simulink model "gm_hybrid_lht_vnl"  (R2019b)
settings: Solver=FixedStepDiscrete  StartTime=0.0  StopTime=inf  FixedStep=1/120e6  RelTol=1e-3
undefined symbols (not defined in the file or in its folder): bt, height, nTheta, width
libraries: hdlsllib x632, simulink x518, hdlmdlgenlib x7, dspsrcs4 x1
(part 7 of 18)

== system gm_hybrid_lht_vnl/Hybrid LHT/Hybrid LHT Accumulator/Accumulator with Switches/Accumulator_instance7 ==
  shift : Inport  OutDataTypeStr=fixdt(0, 6, 0)  PortDimensions=1  SampleTime=8.33333333333333e-09
  mode : Inport  Port=2  OutDataTypeStr=boolean  PortDimensions=1  SampleTime=8.33333333333333e-09
  address : Inport  Port=3  OutDataTypeStr=fixdt(0, 11, 0)  PortDimensions=1  SampleTime=8.33333333333333e-09
  edge : Inport  Port=4  OutDataTypeStr=boolean  PortDimensions=1  SampleTime=8.33333333333333e-09
  AND : Logic  IconShape=distinctive  AllPortsSameDT=off  OutDataTypeStr=boolean
  Add : Sum  OutDataTypeStr=fixdt(0, ceil(log2(maxRho*2)), 0)
  Bit Concat : hdlsllib/Logic and Bit Operations/Bit Concat  numInputs=2
      settings: SourceProductName=Simulink
  Bit Slice : hdlsllib/Logic and Bit Operations/Bit Slice  lidx=voteWL-1  ridx=0
  Bitwise AND : simulink/Logic and Bit Operations/Bitwise Operator  logicop=AND  UseBitMask=off  NumInputPorts=2  BitMask=bin2dec('11011001')  BitMaskRealWorld=Stored Integer
  Bitwise NOT : simulink/Logic and Bit Operations/Bitwise Operator  logicop=NOT  UseBitMask=off  BitMask=bin2dec('11011001')  BitMaskRealWorld=Stored Integer
  Bitwise OR : simulink/Logic and Bit Operations/Bitwise Operator  logicop=OR  UseBitMask=off  NumInputPorts=2  BitMask=bin2dec('11011001')  BitMaskRealWorld=Stored Integer
  Block RAM : Subsystem
  Constant : Constant  Value=0  OutDataTypeStr=fixdt(0, 36-voteWL, 0)  SampleTime=-1
  Constant1 : Constant  Value=2^(voteWL)-1  OutDataTypeStr=fixdt(0, 36, 0)  SampleTime=-1
  Delay{,1..2,4..5} (5 alike) : Delay  DelayLength=1
  Multiport Switch : MultiPortSwitch  DataPortOrder=Zero-based contiguous  Inputs=2  zeroidx=on
  Multiport Switch1 : MultiPortSwitch  DataPortOrder=Zero-based contiguous  Inputs=2  zeroidx=on
  Relational Operator : RelationalOperator  Operator===  OutDataTypeStr=boolean  RndMeth=Simplest
  Shift Arithmetic : ArithShift  BitShiftNumberSource=Input port  BitShiftNumber=8  BitShiftDirection=Left  DiagnosticForOORShift=Error
      settings: InputPortMap=u0,p1
  Shift Arithmetic1 : ArithShift  BitShiftNumberSource=Input port  BitShiftNumber=8  BitShiftDirection=Left  DiagnosticForOORShift=Error
      settings: InputPortMap=u0,p1
  Shift Arithmetic2 : ArithShift  BitShiftNumberSource=Input port  BitShiftNumber=8  BitShiftDirection=Right  DiagnosticForOORShift=Error
      settings: InputPortMap=u0,p1
  Signal Specification : SignalSpecification  OutDataTypeStr=fixdt(0, 36, 0)
  Vote : Constant  OutDataTypeStr=fixdt(0,1,0)  SampleTime=-1
  Zero : Constant  Value=0  OutDataTypeStr=fixdt(0,1,0)  SampleTime=-1
  hps : Outport
  wires:
  Zero/1 -> Multiport Switch/2
  Vote/1 -> Add/1
  Shift Arithmetic1/1 -> Bitwise NOT/1
  Relational Operator/1 -> AND/2
  Delay4/1 -> Shift Arithmetic1/2, Shift Arithmetic/2, Shift Arithmetic2/2
  Delay2/1 -> Multiport Switch1/1
  Delay1/1 -> AND/1, Block RAM/3(wr_en)
  Delay/1 -> Relational Operator/1, Block RAM/2(wr_addr)
  Constant1/1 -> Shift Arithmetic1/1
  Constant/1 -> Bit Concat/1
  Bitwise NOT/1 -> Bitwise AND/1
  Bit Slice/1 -> hps/1, Add/2
  AND/1 -> Delay2/1
  shift/1 -> Delay4/1
  mode/1 -> Multiport Switch/1
  address/1 -> Relational Operator/2, Delay/1, Block RAM/4(rd_addr)
  edge/1 -> Delay1/1
  Delay5/1 -> Multiport Switch1/3
  Shift Arithmetic/1 -> Bitwise OR/2
  Bit Concat/1 -> Shift Arithmetic/1
  Multiport Switch/1 -> Bit Concat/2
  Add/1 -> Multiport Switch/3
  Shift Arithmetic2/1 -> Bit Slice/1
  Bitwise AND/1 -> Bitwise OR/1
  Bitwise OR/1 -> Delay5/1, Block RAM/1(wr_data)
  Signal Specification/1 -> Multiport Switch1/2
  Multiport Switch1/1 -> Bitwise AND/2, Shift Arithmetic2/1
  Block RAM/1(rd_data) -> Signal Specification/1

== system gm_hybrid_lht_vnl/Hybrid LHT/Hybrid LHT Accumulator/Accumulator with Switches/Accumulator_instance8 ==
  shift : Inport  OutDataTypeStr=fixdt(0, 6, 0)  PortDimensions=1  SampleTime=8.33333333333333e-09
  mode : Inport  Port=2  OutDataTypeStr=boolean  PortDimensions=1  SampleTime=8.33333333333333e-09
  address : Inport  Port=3  OutDataTypeStr=fixdt(0, 11, 0)  PortDimensions=1  SampleTime=8.33333333333333e-09
  edge : Inport  Port=4  OutDataTypeStr=boolean  PortDimensions=1  SampleTime=8.33333333333333e-09
  AND : Logic  IconShape=distinctive  AllPortsSameDT=off  OutDataTypeStr=boolean
  Add : Sum  OutDataTypeStr=fixdt(0, ceil(log2(maxRho*2)), 0)
  Bit Concat : hdlsllib/Logic and Bit Operations/Bit Concat  numInputs=2
      settings: SourceProductName=Simulink
  Bit Slice : hdlsllib/Logic and Bit Operations/Bit Slice  lidx=voteWL-1  ridx=0
  Bitwise AND : simulink/Logic and Bit Operations/Bitwise Operator  logicop=AND  UseBitMask=off  NumInputPorts=2  BitMask=bin2dec('11011001')  BitMaskRealWorld=Stored Integer
  Bitwise NOT : simulink/Logic and Bit Operations/Bitwise Operator  logicop=NOT  UseBitMask=off  BitMask=bin2dec('11011001')  BitMaskRealWorld=Stored Integer
  Bitwise OR : simulink/Logic and Bit Operations/Bitwise Operator  logicop=OR  UseBitMask=off  NumInputPorts=2  BitMask=bin2dec('11011001')  BitMaskRealWorld=Stored Integer
  Block RAM : Subsystem
  Constant : Constant  Value=0  OutDataTypeStr=fixdt(0, 36-voteWL, 0)  SampleTime=-1
  Constant1 : Constant  Value=2^(voteWL)-1  OutDataTypeStr=fixdt(0, 36, 0)  SampleTime=-1
  Delay{,1..2,4..5} (5 alike) : Delay  DelayLength=1
  Multiport Switch : MultiPortSwitch  DataPortOrder=Zero-based contiguous  Inputs=2  zeroidx=on
  Multiport Switch1 : MultiPortSwitch  DataPortOrder=Zero-based contiguous  Inputs=2  zeroidx=on
  Relational Operator : RelationalOperator  Operator===  OutDataTypeStr=boolean  RndMeth=Simplest
  Shift Arithmetic : ArithShift  BitShiftNumberSource=Input port  BitShiftNumber=8  BitShiftDirection=Left  DiagnosticForOORShift=Error
      settings: InputPortMap=u0,p1
  Shift Arithmetic1 : ArithShift  BitShiftNumberSource=Input port  BitShiftNumber=8  BitShiftDirection=Left  DiagnosticForOORShift=Error
      settings: InputPortMap=u0,p1
  Shift Arithmetic2 : ArithShift  BitShiftNumberSource=Input port  BitShiftNumber=8  BitShiftDirection=Right  DiagnosticForOORShift=Error
      settings: InputPortMap=u0,p1
  Signal Specification : SignalSpecification  OutDataTypeStr=fixdt(0, 36, 0)
  Vote : Constant  OutDataTypeStr=fixdt(0,1,0)  SampleTime=-1
  Zero : Constant  Value=0  OutDataTypeStr=fixdt(0,1,0)  SampleTime=-1
  hps : Outport
  wires:
  Zero/1 -> Multiport Switch/2
  Vote/1 -> Add/1
  Shift Arithmetic1/1 -> Bitwise NOT/1
  Relational Operator/1 -> AND/2
  Delay4/1 -> Shift Arithmetic1/2, Shift Arithmetic/2, Shift Arithmetic2/2
  Delay2/1 -> Multiport Switch1/1
  Delay1/1 -> AND/1, Block RAM/3(wr_en)
  Delay/1 -> Relational Operator/1, Block RAM/2(wr_addr)
  Constant1/1 -> Shift Arithmetic1/1
  Constant/1 -> Bit Concat/1
  Bitwise NOT/1 -> Bitwise AND/1
  Bit Slice/1 -> hps/1, Add/2
  AND/1 -> Delay2/1
  shift/1 -> Delay4/1
  mode/1 -> Multiport Switch/1
  address/1 -> Relational Operator/2, Delay/1, Block RAM/4(rd_addr)
  edge/1 -> Delay1/1
  Delay5/1 -> Multiport Switch1/3
  Shift Arithmetic/1 -> Bitwise OR/2
  Bit Concat/1 -> Shift Arithmetic/1
  Multiport Switch/1 -> Bit Concat/2
  Add/1 -> Multiport Switch/3
  Shift Arithmetic2/1 -> Bit Slice/1
  Bitwise AND/1 -> Bitwise OR/1
  Bitwise OR/1 -> Delay5/1, Block RAM/1(wr_data)
  Signal Specification/1 -> Multiport Switch1/2
  Multiport Switch1/1 -> Bitwise AND/2, Shift Arithmetic2/1
  Block RAM/1(rd_data) -> Signal Specification/1

== system gm_hybrid_lht_vnl/Hybrid LHT/Hybrid LHT Accumulator/Accumulator with Switches/Accumulator_instance9 ==
  shift : Inport  OutDataTypeStr=fixdt(0, 6, 0)  PortDimensions=1  SampleTime=8.33333333333333e-09
  mode : Inport  Port=2  OutDataTypeStr=boolean  PortDimensions=1  SampleTime=8.33333333333333e-09
  address : Inport  Port=3  OutDataTypeStr=fixdt(0, 11, 0)  PortDimensions=1  SampleTime=8.33333333333333e-09
  edge : Inport  Port=4  OutDataTypeStr=boolean  PortDimensions=1  SampleTime=8.33333333333333e-09
  AND : Logic  IconShape=distinctive  AllPortsSameDT=off  OutDataTypeStr=boolean
  Add : Sum  OutDataTypeStr=fixdt(0, ceil(log2(maxRho*2)), 0)
  Bit Concat : hdlsllib/Logic and Bit Operations/Bit Concat  numInputs=2
      settings: SourceProductName=Simulink
  Bit Slice : hdlsllib/Logic and Bit Operations/Bit Slice  lidx=voteWL-1  ridx=0
  Bitwise AND : simulink/Logic and Bit Operations/Bitwise Operator  logicop=AND  UseBitMask=off  NumInputPorts=2  BitMask=bin2dec('11011001')  BitMaskRealWorld=Stored Integer
  Bitwise NOT : simulink/Logic and Bit Operations/Bitwise Operator  logicop=NOT  UseBitMask=off  BitMask=bin2dec('11011001')  BitMaskRealWorld=Stored Integer
  Bitwise OR : simulink/Logic and Bit Operations/Bitwise Operator  logicop=OR  UseBitMask=off  NumInputPorts=2  BitMask=bin2dec('11011001')  BitMaskRealWorld=Stored Integer
  Block RAM : Subsystem
  Constant : Constant  Value=0  OutDataTypeStr=fixdt(0, 36-voteWL, 0)  SampleTime=-1
  Constant1 : Constant  Value=2^(voteWL)-1  OutDataTypeStr=fixdt(0, 36, 0)  SampleTime=-1
  Delay{,1..2,4..5} (5 alike) : Delay  DelayLength=1
  Multiport Switch : MultiPortSwitch  DataPortOrder=Zero-based contiguous  Inputs=2  zeroidx=on
  Multiport Switch1 : MultiPortSwitch  DataPortOrder=Zero-based contiguous  Inputs=2  zeroidx=on
  Relational Operator : RelationalOperator  Operator===  OutDataTypeStr=boolean  RndMeth=Simplest
  Shift Arithmetic : ArithShift  BitShiftNumberSource=Input port  BitShiftNumber=8  BitShiftDirection=Left  DiagnosticForOORShift=Error
      settings: InputPortMap=u0,p1
  Shift Arithmetic1 : ArithShift  BitShiftNumberSource=Input port  BitShiftNumber=8  BitShiftDirection=Left  DiagnosticForOORShift=Error
      settings: InputPortMap=u0,p1
  Shift Arithmetic2 : ArithShift  BitShiftNumberSource=Input port  BitShiftNumber=8  BitShiftDirection=Right  DiagnosticForOORShift=Error
      settings: InputPortMap=u0,p1
  Signal Specification : SignalSpecification  OutDataTypeStr=fixdt(0, 36, 0)
  Vote : Constant  OutDataTypeStr=fixdt(0,1,0)  SampleTime=-1
  Zero : Constant  Value=0  OutDataTypeStr=fixdt(0,1,0)  SampleTime=-1
  hps : Outport
  wires:
  Zero/1 -> Multiport Switch/2
  Vote/1 -> Add/1
  Shift Arithmetic1/1 -> Bitwise NOT/1
  Relational Operator/1 -> AND/2
  Delay4/1 -> Shift Arithmetic1/2, Shift Arithmetic/2, Shift Arithmetic2/2
  Delay2/1 -> Multiport Switch1/1
  Delay1/1 -> AND/1, Block RAM/3(wr_en)
  Delay/1 -> Relational Operator/1, Block RAM/2(wr_addr)
  Constant1/1 -> Shift Arithmetic1/1
  Constant/1 -> Bit Concat/1
  Bitwise NOT/1 -> Bitwise AND/1
  Bit Slice/1 -> hps/1, Add/2
  AND/1 -> Delay2/1
  shift/1 -> Delay4/1
  mode/1 -> Multiport Switch/1
  address/1 -> Relational Operator/2, Delay/1, Block RAM/4(rd_addr)
  edge/1 -> Delay1/1
  Delay5/1 -> Multiport Switch1/3
  Shift Arithmetic/1 -> Bitwise OR/2
  Bit Concat/1 -> Shift Arithmetic/1
  Multiport Switch/1 -> Bit Concat/2
  Add/1 -> Multiport Switch/3
  Shift Arithmetic2/1 -> Bit Slice/1
  Bitwise AND/1 -> Bitwise OR/1
  Bitwise OR/1 -> Delay5/1, Block RAM/1(wr_data)
  Signal Specification/1 -> Multiport Switch1/2
  Multiport Switch1/1 -> Bitwise AND/2, Shift Arithmetic2/1
  Block RAM/1(rd_data) -> Signal Specification/1

== system gm_hybrid_lht_vnl/Hybrid LHT/Hybrid LHT Kernel/Extract Active Votes/GetShift ==
  Theta : Inport  OutDataTypeStr=uint8  PortDimensions=1  SampleTime=8.33333333333333e-09
  Add : Sum  Inputs=+  OutDataTypeStr=fixdt(0, ceil(log2(L+1)), 0)
  Constant : Constant  Value=U  VectorParams1D=off  OutDataTypeStr=fixdt(0,ceil(log2(max(U)+1)),0)  SampleTime=-1
  Relational Operator : RelationalOperator  OutDataTypeStr=boolean  RndMeth=Nearest
  Shift : Outport  VectorParamsAs1DForOutWhenUnconnected=off
  wires:
  Theta/1 -> Relational Operator/1
  Relational Operator/1 -> Add/1
  Constant/1 -> Relational Operator/2
  Add/1 -> Shift/1

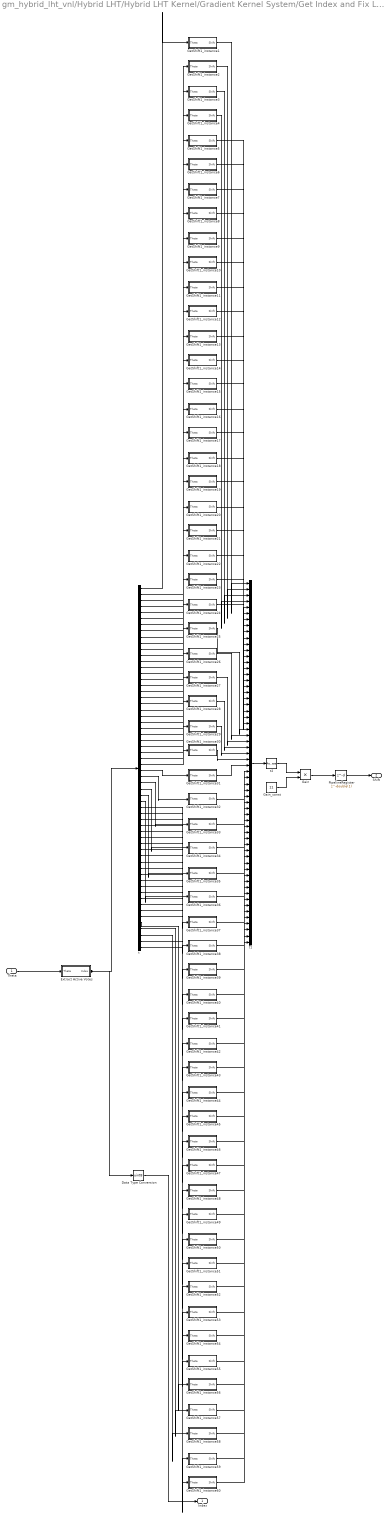
== system gm_hybrid_lht_vnl/Hybrid LHT/Hybrid LHT Kernel/Gradient Kernel System/Get Index and Fix Limits ==
  Theta : Inport  OutDataTypeStr=uint8  PortDimensions=1  SampleTime=8.33333333333333e-09
  Data Type Conversion : DataTypeConversion  OutDataTypeStr=uint8  SampleTime=8.33333333333333e-09
  Extract Active Votes : Subsystem
  Gain : Product  Inputs=**  OutDataTypeStr=fixdt(0, 6, 0)  SampleTime=8.33333333333333e-09
  Gain_const : Constant  Value=11  OutDataTypeStr=fixdt(0, 6, 0)  SampleTime=-1
  GetShift1_instance1 : Subsystem
  GetShift1_instance10 : Subsystem
  GetShift1_instance11 : Subsystem
  GetShift1_instance12 : Subsystem
  GetShift1_instance13 : Subsystem
  GetShift1_instance14 : Subsystem
  GetShift1_instance15 : Subsystem
  GetShift1_instance16 : Subsystem
  GetShift1_instance17 : Subsystem
  GetShift1_instance18 : Subsystem
  GetShift1_instance19 : Subsystem
  GetShift1_instance2 : Subsystem
  GetShift1_instance20 : Subsystem
  GetShift1_instance21 : Subsystem
  GetShift1_instance22 : Subsystem
  GetShift1_instance23 : Subsystem
  GetShift1_instance24 : Subsystem
  GetShift1_instance25 : Subsystem
  GetShift1_instance26 : Subsystem
  GetShift1_instance27 : Subsystem
  GetShift1_instance28 : Subsystem
  GetShift1_instance29 : Subsystem
  GetShift1_instance3 : Subsystem
  GetShift1_instance30 : Subsystem
  GetShift1_instance31 : Subsystem
  GetShift1_instance32 : Subsystem
  GetShift1_instance33 : Subsystem
  GetShift1_instance34 : Subsystem
  GetShift1_instance35 : Subsystem
  GetShift1_instance36 : Subsystem
  GetShift1_instance37 : Subsystem
  GetShift1_instance38 : Subsystem
  GetShift1_instance39 : Subsystem
  GetShift1_instance4 : Subsystem
  GetShift1_instance40 : Subsystem
  GetShift1_instance41 : Subsystem
  GetShift1_instance42 : Subsystem
  GetShift1_instance43 : Subsystem
  GetShift1_instance44 : Subsystem
  GetShift1_instance45 : Subsystem
  GetShift1_instance46 : Subsystem
  GetShift1_instance47 : Subsystem
  GetShift1_instance48 : Subsystem
  GetShift1_instance49 : Subsystem
  GetShift1_instance5 : Subsystem
  GetShift1_instance50 : Subsystem
  GetShift1_instance51 : Subsystem
  GetShift1_instance52 : Subsystem
  GetShift1_instance53 : Subsystem
  GetShift1_instance54 : Subsystem
  GetShift1_instance55 : Subsystem
  GetShift1_instance56 : Subsystem
  GetShift1_instance57 : Subsystem
  GetShift1_instance58 : Subsystem
  GetShift1_instance59 : Subsystem
  GetShift1_instance6 : Subsystem
  GetShift1_instance60 : Subsystem
  GetShift1_instance7 : Subsystem
  GetShift1_instance8 : Subsystem
  GetShift1_instance9 : Subsystem
  PipelineRegister : Delay  DelayLength=double(1)  InitialCondition=0  SampleTime=8.33333333333333e-09
  t : Demux  Outputs=60
  t1 : Concatenate  NumInputs=60
  t2 : Reshape  OutputDimensionality=Row vector (2-D)
  Index : Outport  VectorParamsAs1DForOutWhenUnconnected=off
  Shift : Outport  Port=2  VectorParamsAs1DForOutWhenUnconnected=off
  wires:
  Gain/1 -> PipelineRegister/1
  Theta/1 -> Extract Active Votes/1(Theta)
  Gain_const/1 -> Gain/2
  GetShift1_instance60/1(Shift) -> t1/60
  GetShift1_instance59/1(Shift) -> t1/59
  GetShift1_instance58/1(Shift) -> t1/58
  GetShift1_instance57/1(Shift) -> t1/57
  GetShift1_instance56/1(Shift) -> t1/56
  GetShift1_instance55/1(Shift) -> t1/55
  GetShift1_instance54/1(Shift) -> t1/54
  GetShift1_instance53/1(Shift) -> t1/53
  GetShift1_instance52/1(Shift) -> t1/52
  GetShift1_instance51/1(Shift) -> t1/51
  GetShift1_instance50/1(Shift) -> t1/50
  GetShift1_instance49/1(Shift) -> t1/49
  GetShift1_instance48/1(Shift) -> t1/48
  GetShift1_instance47/1(Shift) -> t1/47
  GetShift1_instance46/1(Shift) -> t1/46
  GetShift1_instance45/1(Shift) -> t1/45
  GetShift1_instance44/1(Shift) -> t1/44
  GetShift1_instance43/1(Shift) -> t1/43
  GetShift1_instance42/1(Shift) -> t1/42
  GetShift1_instance41/1(Shift) -> t1/41
  GetShift1_instance40/1(Shift) -> t1/40
  GetShift1_instance39/1(Shift) -> t1/39
  GetShift1_instance38/1(Shift) -> t1/38
  GetShift1_instance37/1(Shift) -> t1/37
  GetShift1_instance36/1(Shift) -> t1/36
  GetShift1_instance35/1(Shift) -> t1/35
  GetShift1_instance34/1(Shift) -> t1/34
  GetShift1_instance33/1(Shift) -> t1/33
  GetShift1_instance32/1(Shift) -> t1/32
  GetShift1_instance31/1(Shift) -> t1/31
  GetShift1_instance30/1(Shift) -> t1/30
  GetShift1_instance29/1(Shift) -> t1/29
  GetShift1_instance28/1(Shift) -> t1/28
  GetShift1_instance27/1(Shift) -> t1/27
  GetShift1_instance26/1(Shift) -> t1/26
  GetShift1_instance25/1(Shift) -> t1/25
  GetShift1_instance24/1(Shift) -> t1/24
  GetShift1_instance23/1(Shift) -> t1/23
  GetShift1_instance22/1(Shift) -> t1/22
  GetShift1_instance21/1(Shift) -> t1/21
  GetShift1_instance20/1(Shift) -> t1/20
  GetShift1_instance19/1(Shift) -> t1/19
  GetShift1_instance18/1(Shift) -> t1/18
  GetShift1_instance17/1(Shift) -> t1/17
  GetShift1_instance16/1(Shift) -> t1/16
  GetShift1_instance15/1(Shift) -> t1/15
  GetShift1_instance14/1(Shift) -> t1/14
  GetShift1_instance13/1(Shift) -> t1/13
  GetShift1_instance12/1(Shift) -> t1/12
  GetShift1_instance11/1(Shift) -> t1/11
  GetShift1_instance10/1(Shift) -> t1/10
  GetShift1_instance9/1(Shift) -> t1/9
  GetShift1_instance8/1(Shift) -> t1/8
  GetShift1_instance7/1(Shift) -> t1/7
  GetShift1_instance6/1(Shift) -> t1/6
  GetShift1_instance5/1(Shift) -> t1/5
  GetShift1_instance4/1(Shift) -> t1/4
  GetShift1_instance3/1(Shift) -> t1/3
  GetShift1_instance2/1(Shift) -> t1/2
  GetShift1_instance1/1(Shift) -> t1/1
  t1/1 -> t2/1
  t/60 -> GetShift1_instance60/1(Theta)
  t/59 -> GetShift1_instance59/1(Theta)
  t/58 -> GetShift1_instance58/1(Theta)
  t/57 -> GetShift1_instance57/1(Theta)
  t/56 -> GetShift1_instance56/1(Theta)
  t/55 -> GetShift1_instance55/1(Theta)
  t/54 -> GetShift1_instance54/1(Theta)
  t/53 -> GetShift1_instance53/1(Theta)
  t/52 -> GetShift1_instance52/1(Theta)
  t/51 -> GetShift1_instance51/1(Theta)
  t/50 -> GetShift1_instance50/1(Theta)
  t/49 -> GetShift1_instance49/1(Theta)
  t/48 -> GetShift1_instance48/1(Theta)
  t/47 -> GetShift1_instance47/1(Theta)
  t/46 -> GetShift1_instance46/1(Theta)
  t/45 -> GetShift1_instance45/1(Theta)
  t/44 -> GetShift1_instance44/1(Theta)
  t/43 -> GetShift1_instance43/1(Theta)
  t/42 -> GetShift1_instance42/1(Theta)
  t/41 -> GetShift1_instance41/1(Theta)
  t/40 -> GetShift1_instance40/1(Theta)
  t/39 -> GetShift1_instance39/1(Theta)
  t/38 -> GetShift1_instance38/1(Theta)
  t/37 -> GetShift1_instance37/1(Theta)
  t/36 -> GetShift1_instance36/1(Theta)
  t/35 -> GetShift1_instance35/1(Theta)
  t/34 -> GetShift1_instance34/1(Theta)
  t/33 -> GetShift1_instance33/1(Theta)
  t/32 -> GetShift1_instance32/1(Theta)
  t/31 -> GetShift1_instance31/1(Theta)
  t/30 -> GetShift1_instance30/1(Theta)
  t/29 -> GetShift1_instance29/1(Theta)
  t/28 -> GetShift1_instance28/1(Theta)
  t/27 -> GetShift1_instance27/1(Theta)
  t/26 -> GetShift1_instance26/1(Theta)
  t/25 -> GetShift1_instance25/1(Theta)
  t/24 -> GetShift1_instance24/1(Theta)
  t/23 -> GetShift1_instance23/1(Theta)
  t/22 -> GetShift1_instance22/1(Theta)
  t/21 -> GetShift1_instance21/1(Theta)
  t/20 -> GetShift1_instance20/1(Theta)
  t/19 -> GetShift1_instance19/1(Theta)
  t/18 -> GetShift1_instance18/1(Theta)
  t/17 -> GetShift1_instance17/1(Theta)
  t/16 -> GetShift1_instance16/1(Theta)
  t/15 -> GetShift1_instance15/1(Theta)
  t/14 -> GetShift1_instance14/1(Theta)
  t/13 -> GetShift1_instance13/1(Theta)
  t/12 -> GetShift1_instance12/1(Theta)
  t/11 -> GetShift1_instance11/1(Theta)
  t/10 -> GetShift1_instance10/1(Theta)
  t/9 -> GetShift1_instance9/1(Theta)
  t/8 -> GetShift1_instance8/1(Theta)
  t/7 -> GetShift1_instance7/1(Theta)
  t/6 -> GetShift1_instance6/1(Theta)
  t/5 -> GetShift1_instance5/1(Theta)
  t/4 -> GetShift1_instance4/1(Theta)
  t/3 -> GetShift1_instance3/1(Theta)
  t/2 -> GetShift1_instance2/1(Theta)
  t/1 -> GetShift1_instance1/1(Theta)
  t2/1 -> Gain/1
  PipelineRegister/1 -> Shift/1
  Extract Active Votes/1(Index) -> t/1, Data Type Conversion/1
  Data Type Conversion/1 -> Index/1

== system gm_hybrid_lht_vnl/Hybrid LHT/Hybrid LHT Kernel/Gradient Kernel System/Hough Kernel ==
  Edge : Inport  OutDataTypeStr=fixdt(0, 1, 0)  PortDimensions=1  SampleTime=8.33333333333333e-09
  X : Inport  Port=2  OutDataTypeStr=fixdt(1, 10, 0)  PortDimensions=1  SampleTime=8.33333333333333e-09
  Y : Inport  Port=3  OutDataTypeStr=fixdt(1, 10, 0)  PortDimensions=1  SampleTime=8.33333333333333e-09
  Index : Inport  Port=4  OutDataTypeStr=uint8  PortDimensions=[1 60]  SampleTime=8.33333333333333e-09
  Add1 : Sum  OutDataTypeStr=fixdt(0, ceil(log2(2*maxRho)), 0)  RndMeth=Round
  Compare To Constant1 : simulink/Logic and Bit Operations/Compare To Constant  relop===  const=width/2-1  OutDataTypeStr=boolean
  Constant : Constant  Value=maxRho  OutDataTypeStr=fixdt(0, ceil(log2(maxRho + 1)), 0);  SampleTime=-1
  Data Type Conversion : DataTypeConversion  OutDataTypeStr=uint8
  Hough Kernel : Subsystem
  Look Ahead Hough : Subsystem
  vEdge : Outport  VectorParamsAs1DForOutWhenUnconnected=off
  Rho : Outport  Port=2  VectorParamsAs1DForOutWhenUnconnected=off
  wires:
  Index/1 -> Data Type Conversion/1
  Y/1 -> Look Ahead Hough/1(Y)
  X/1 -> Hough Kernel/1(X), Compare To Constant1/1
  Edge/1 -> vEdge/1
  Look Ahead Hough/1(ysin) -> Hough Kernel/2(Y)
  Hough Kernel/1(Rho) -> Add1/1
  Data Type Conversion/1 -> Hough Kernel/3(Index)
  Constant/1 -> Add1/2
  Compare To Constant1/1 -> Look Ahead Hough/2(eol)
  Add1/1 -> Rho/1

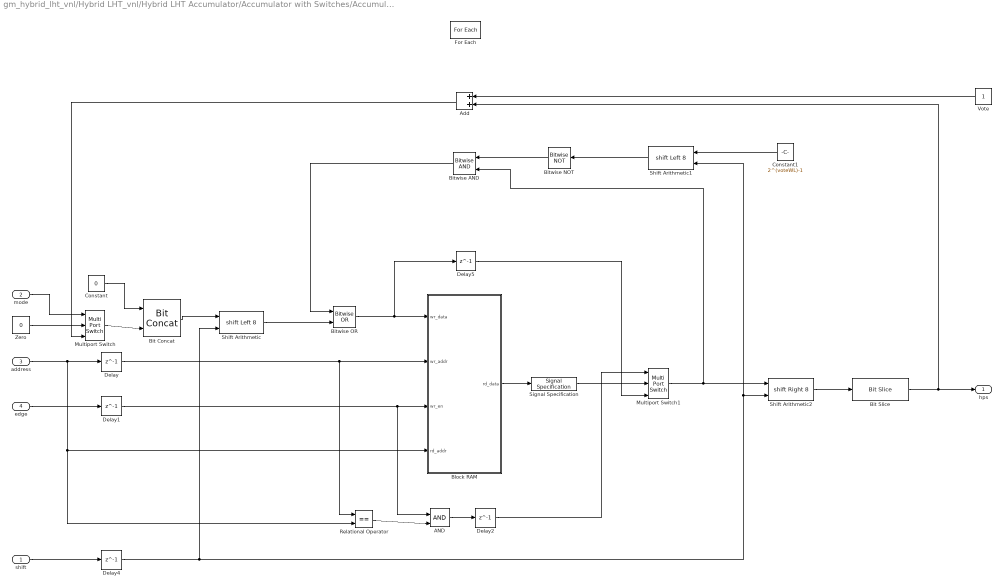
== system gm_hybrid_lht_vnl/Hybrid LHT_vnl/Hybrid LHT Accumulator/Accumulator with Switches/Accumulator ==
  shift : Inport  Partition=on  PartitionDimension=2  PartitionWidth=1  PartitionOffset=0
  mode : Inport  Port=2
  address : Inport  Port=3  Partition=on  PartitionDimension=2  PartitionWidth=1  PartitionOffset=0
  edge : Inport  Port=4
  AND : Logic  IconShape=distinctive  AllPortsSameDT=off  OutDataTypeStr=boolean
  Add : Sum  OutDataTypeStr=fixdt(0, ceil(log2(maxRho*2)), 0)
  Bit Concat : hdlsllib/Logic and Bit Operations/Bit Concat  numInputs=2
      settings: SourceProductName=Simulink
  Bit Slice : hdlsllib/Logic and Bit Operations/Bit Slice  lidx=voteWL-1  ridx=0
  Bitwise AND : simulink/Logic and Bit Operations/Bitwise Operator  logicop=AND  UseBitMask=off  NumInputPorts=2  BitMask=bin2dec('11011001')  BitMaskRealWorld=Stored Integer
  Bitwise NOT : simulink/Logic and Bit Operations/Bitwise Operator  logicop=NOT  UseBitMask=off  BitMask=bin2dec('11011001')  BitMaskRealWorld=Stored Integer
  Bitwise OR : simulink/Logic and Bit Operations/Bitwise Operator  logicop=OR  UseBitMask=off  NumInputPorts=2  BitMask=bin2dec('11011001')  BitMaskRealWorld=Stored Integer
  Block RAM : Subsystem  VariantControlMode=Label  Variant=on  VariantControl=Variant1  LabelModeActiveChoice=other_bits
  Constant : Constant  Value=0  OutDataTypeStr=fixdt(0, 36-voteWL, 0)  SampleTime=-1
  Constant1 : Constant  Value=2^(voteWL)-1  OutDataTypeStr=fixdt(0, 36, 0)  SampleTime=-1
  Delay{,1..2,4..5} (5 alike) : Delay  DelayLength=1
  For Each : ForEach  DisableCoverage=on
  Multiport Switch : MultiPortSwitch  DataPortOrder=Zero-based contiguous  Inputs=2  zeroidx=on
  Multiport Switch1 : MultiPortSwitch  DataPortOrder=Zero-based contiguous  Inputs=2  zeroidx=on
  Relational Operator : RelationalOperator  Operator===  OutDataTypeStr=boolean  RndMeth=Simplest
  Shift Arithmetic : ArithShift  BitShiftNumberSource=Input port  BitShiftNumber=8  BitShiftDirection=Left  DiagnosticForOORShift=Error
      settings: InputPortMap=u0,p1
  Shift Arithmetic1 : ArithShift  BitShiftNumberSource=Input port  BitShiftNumber=8  BitShiftDirection=Left  DiagnosticForOORShift=Error
      settings: InputPortMap=u0,p1
  Shift Arithmetic2 : ArithShift  BitShiftNumberSource=Input port  BitShiftNumber=8  BitShiftDirection=Right  DiagnosticForOORShift=Error
      settings: InputPortMap=u0,p1
  Signal Specification : SignalSpecification  OutDataTypeStr=fixdt(0, 36, 0)
  Vote : Constant  OutDataTypeStr=fixdt(0,1,0)  SampleTime=-1
  Zero : Constant  Value=0  OutDataTypeStr=fixdt(0,1,0)  SampleTime=-1
  hps : Outport  ConcatenationDimension=2
  wires:
  Bitwise NOT/1 -> Bitwise AND/1
  Multiport Switch1/1 -> Shift Arithmetic2/1, Bitwise AND/2
  Delay5/1 -> Multiport Switch1/3
  Bit Slice/1 -> hps/1, Add/2
  Shift Arithmetic2/1 -> Bit Slice/1
  Signal Specification/1 -> Multiport Switch1/2
  Constant1/1 -> Shift Arithmetic1/1
  Shift Arithmetic1/1 -> Bitwise NOT/1
  Bitwise OR/1 -> Block RAM/1(wr_data), Delay5/1
  Bitwise AND/1 -> Bitwise OR/1
  Shift Arithmetic/1 -> Bitwise OR/2
  Delay4/1 -> Shift Arithmetic/2, Shift Arithmetic2/2, Shift Arithmetic1/2
  shift/1 -> Delay4/1
  Bit Concat/1 -> Shift Arithmetic/1
  Constant/1 -> Bit Concat/1
  Multiport Switch/1 -> Bit Concat/2
  Relational Operator/1 -> AND/2
  Delay/1 -> Relational Operator/1, Block RAM/2(wr_addr)
  Delay2/1 -> Multiport Switch1/1
  address/1 -> Delay/1, Relational Operator/2, Block RAM/4(rd_addr)
  AND/1 -> Delay2/1
  Delay1/1 -> AND/1, Block RAM/3(wr_en)
  Add/1 -> Multiport Switch/3
  Vote/1 -> Add/1
  Zero/1 -> Multiport Switch/2
  edge/1 -> Delay1/1
  mode/1 -> Multiport Switch/1
  Block RAM/1(rd_data) -> Signal Specification/1

== system gm_hybrid_lht_vnl/Hybrid LHT_vnl/Hybrid LHT Kernel/Extract Active Votes/GetShift ==
  Theta : Inport
  Add : Sum  Inputs=+  OutDataTypeStr=fixdt(0, ceil(log2(L+1)), 0)
  Constant : Constant  Value=U  VectorParams1D=off  OutDataTypeStr=fixdt(0,ceil(log2(max(U)+1)),0)  SampleTime=-1
  Relational Operator : RelationalOperator  OutDataTypeStr=boolean  RndMeth=Nearest
  Shift : Outport  VectorParamsAs1DForOutWhenUnconnected=off
  wires:
  Relational Operator/1 -> Add/1
  Add/1 -> Shift/1
  Theta/1 -> Relational Operator/1
  Constant/1 -> Relational Operator/2

== system gm_hybrid_lht_vnl/Hybrid LHT_vnl/Hybrid LHT Kernel/Gradient Kernel System/Get Index and Fix Limits ==
  Theta : Inport
  Data Type Conversion : DataTypeConversion  OutDataTypeStr=uint8
  Extract Active Votes : Subsystem
  Gain : Gain  Gain=fi(voteWL, 0, 6, 0)  ParamDataTypeStr=fixdt(0,6,0)  OutDataTypeStr=fixdt(0, 6, 0)
  GetShift1 : Subsystem
  Index : Outport  VectorParamsAs1DForOutWhenUnconnected=off
  Shift : Outport  Port=2  VectorParamsAs1DForOutWhenUnconnected=off
  wires:
  Gain/1 -> Shift/1
  Extract Active Votes/1(Index) -> GetShift1/1(Theta), Data Type Conversion/1
  Theta/1 -> Extract Active Votes/1(Theta)
  Data Type Conversion/1 -> Index/1
  GetShift1/1(Shift) -> Gain/1

== system gm_hybrid_lht_vnl/Hybrid LHT_vnl/Hybrid LHT Kernel/Gradient Kernel System/Hough Kernel ==
  Edge : Inport
  X : Inport  Port=2
  Y : Inport  Port=3
  Index : Inport  Port=4
  Add1 : Sum  OutDataTypeStr=fixdt(0, ceil(log2(2*maxRho)), 0)  RndMeth=Round
  Compare To Constant1 : simulink/Logic and Bit Operations/Compare To Constant  relop===  const=width/2-1  OutDataTypeStr=boolean
  Constant : Constant  Value=maxRho  OutDataTypeStr=fixdt(0, ceil(log2(maxRho + 1)), 0);  SampleTime=-1
  Data Type Conversion : DataTypeConversion  OutDataTypeStr=uint8
  Hough Kernel : Subsystem
  Look Ahead Hough : Subsystem  VariantControlMode=Label  Variant=on  VariantControl=Variant1  LabelModeActiveChoice=Symmetric
  vEdge : Outport  VectorParamsAs1DForOutWhenUnconnected=off
  Rho : Outport  Port=2  VectorParamsAs1DForOutWhenUnconnected=off
  wires:
  Look Ahead Hough/1(ysin) -> Hough Kernel/2(Y)
  Compare To Constant1/1 -> Look Ahead Hough/2(eol)
  Y/1 -> Look Ahead Hough/1(Y)
  X/1 -> Hough Kernel/1(X), Compare To Constant1/1
  Edge/1 -> vEdge/1
  Hough Kernel/1(Rho) -> Add1/1
  Data Type Conversion/1 -> Hough Kernel/3(Index)
  Index/1 -> Data Type Conversion/1
  Add1/1 -> Rho/1
  Constant/1 -> Add1/2

== system gm_hybrid_lht_vnl/Hybrid LHT/Hybrid LHT Accumulator/Accumulator with Switches/Accumulator_instance1/Block RAM ==
  wr_data : Inport  OutDataTypeStr=fixdt(0, 36, 0)  PortDimensions=1  SampleTime=8.33333333333333e-09
  wr_addr : Inport  Port=2  OutDataTypeStr=fixdt(0, 11, 0)  PortDimensions=1  SampleTime=8.33333333333333e-09
  wr_en : Inport  Port=3  OutDataTypeStr=boolean  PortDimensions=1  SampleTime=8.33333333333333e-09
  rd_addr : Inport  Port=4  OutDataTypeStr=fixdt(0, 11, 0)  PortDimensions=1  SampleTime=8.33333333333333e-09
  Simple Dual Port RAM Generator : Subsystem  mask{b=double(36), d=double(1280), b_hidden=double(36), d_hidden=double(1280)}
      mask prompts: b "Data width:"; d "Depth:"
      mask init:
      | if d == d_hidden
      |     return
      | end
      | 
      | set_param(gcb, 'd_hidden', int2str(d));
      | 
      | % Xilinx RAM Initialisation
      | xl_config = [512, 72;
      |             1024, 36;
      |             2048, 18;
      |             4096, 9;
      |             8192, 4;
      |             16384, 2;
      |             32768, 1];
      | 
      | % Get length of Xilinx Configuration
      | sizeram = size(xl_config);
      |         
      | % Get the RAM Configuration based on the data width
      | for i = 1:sizeram(1)
      |     if b <= xl_config(i, 2)
      |         a = xl_config(i, :);
      |     end
      | end
      | 
      | % Get number of BRAM required (including half BRAM)
      | numbram = ceil((d/a(1))/0.5)*0.5;
      | fullbram = floor(numbram); % Integer
      | halfbram = (numbram-floor(numbram)) ~= 0; % Boolean
      | 
      | % Get all blocks and delete everything excepts ports
      | H = get(find_system(gcb, 'FindAll', 'on', 'type', 'block'));
      | todelete = setdiff(strcat(repmat({[gcb '/']}, numel(H.Blocks), 1),  H.Blocks),...
      |     strcat(repmat({[gcb '/']}, 5, 1),...
      |     {'wr_data'; 'wr_addr'; 'wr_en'; 'rd_addr'; 'rd_data'}));
      | delete_block(todelete);
      | 
      | % Delete lines
      | for i = 1:numel(H.Lines)
      |     delete_line(H.Lines(i).Handle)
      | end
      | 
      | % Generate full BRAMs
      | y = 0;
      | 
      | % If there is only one ram then the write enable should be directly
      | % connected to the first ram write enable. Else, the write address must be sliced
      | % and the upper bound (over a(2)) compared to zero. This will indicate if
      | % the first ram is the one to be written/read from.
      | 
      | % Common to both implementations
      | % Write Address Slice
      | add_block('hdlsllib/Logic and Bit Operations/Bit Slice',...
      |         [gcb, '/wr_address'], 'Position',...
      |         [160 130 250 170]);
      | % Set bitslice parameters
      | set_param([gcb, '/wr_address'],...
      |     'lidx', int2str(log2(a(1))-1));
      | set_param([gcb, '/wr_address'],...
      |     'ridx', int2str(0));
      | 
      | % Read Address Slice
      | add_block('hdlsllib/Logic and Bit Operations/Bit Slice',...
      |         [gcb, '/rd_address'], 'Position',...
      |         [160 330 250 370]);
      | % Set bitslice parameters
      | set_param([gcb, '/rd_address'],...
      |     'lidx', int2str(log2(a(1))-1));
      | set_param([gcb, '/rd_address'],...
      |     'ridx', int2str(0));
      | 
      | if ceil(numbram) == 1
      |     
      |     i = 1;
      |     
      |     % Add Simple RAM
      |     add_block('hdlsllib/HDL RAMs/Simple Dual Port RAM',...
      |         [gcb, '/simple_ram_', int2str(i-1)], 'Position',...
      |         [635 0+600*y 635+200 400+600*y]);
      | 
      |     % Set RAM parameters
      |     set_param([gcb, '/simple_ram_', int2str(i-1)],...
      |         'ram_size', int2str(log2(a(1))));
      | 
      |     % Connect "wr_data" to "simple_ram_i"
      |     add_line(gcb, ['wr_data/1'], ['simple_ram_', int2str(i-1), '/1'],...
      |         'autorouting', 'on');
      |     
      |     % Connect "wr_addr" to "wr_address"
      |     add_line(gcb, ['wr_addr/1'], ['wr_address/1'],...
      |         'autorouting', 'on');
      | 
      |     % Connect "wr_address" to "simple_ram_i"
      |     add_line(gcb, ['wr_address/1'], ['simple_ram_', int2str(i-1), '/2'],...
      |         'autorouting', 'on');
      | 
      |     % Connect "wr_en" to "simple_ram_i"
      |     add_line(gcb, ['wr_en/1'], ['simple_ram_', int2str(i-1), '/3'],...
      |         'autorouting', 'on');
      |     
      |     % Connect "rd_addr" to "rd_address"
      |     add_line(gcb, ['rd_addr/1'], ['rd_address/1'],...
      |         'autorouting', 'on');
      | 
      |     % Connect "rd_address" to "simple_ram_i"
      |     add_line(gcb, ['rd_address/1'], ['simple_ram_', int2str(i-1), '/4'],...
      |         'autorouting', 'on');
      | 
      |     % Connect "simple_ram_i" to "rd_data"
      |     add_line(gcb, ['simple_ram_', int2str(i-1), '/1'], ['rd_data/1'],...
      |         'autorouting', 'on');
      | 
      | else
      |     
      |     % Multiport Switch
      |     add_block('hdlsllib/Signal Routing/Multiport Switch',...
      |         [gcb, '/multiport_switch'], 'Position',...
      |         [1340 146 1405 250]);
      |     % Set multiport switch parameters
      |     set_param([gcb, '/multiport_switch'],...
      |         'Inputs', int2str(ceil(numbram)));
      |     set_param([gcb, '/multiport_switch'],...
      |         'DataPortOrder', 'Zero-based contiguous');
      | 
      |     % Add Constant Zero
      |     add_block('hdlsllib/Sources/Constant',...
      |         [gcb, '/zero'], 'Position',...
      |         [425 -65 455 -35]);
      |     set_param([gcb, '/zero'],...
      |         'Value', int2str(0));
      |     set_param([gcb, '/zero'],...
      |         'OutDataTypeStr', ['fixdt(0, ', int2str(ceil(numbram)), ', 0)']);
      | 
      |     % Add Vector Concatenate
      |     add_block('hdlsllib/Signal Routing/Vector Concatenate',...
      |         [gcb, '/vector_concatenate'], 'Position',...
      |         [1015, -113, 1025, 38]);
      |     set_param([gcb, '/vector_concatenate'],...
      |         'NumInputs', int2str(ceil(numbram)));
      | 
      |     % Add Bitwise-OR
      |     add_block('hdlsllib/Logic and Bit Operations/Bitwise Operator',...
      |         [gcb, '/bitwise_or'], 'Position',...
      |         [1165, -54, 1205, -16]);
      |     set_param([gcb, '/bitwise_or'],...
      |         'logicop', 'OR');
      |     set_param([gcb, '/bitwise_or'],...
      |         'UseBitMask', 0);
      |     set_param([gcb, '/bitwise_or'],...
      |         'NumInputPorts', int2str(1));
      | 
      |     % Add delay for bram access
      |     add_block('hdlsllib/Discrete/Delay',...
      |         [gcb, '/delay'], 'Position',...
      |         [1248, 60, 1282, 95]);
      |     set_param([gcb, '/delay'],...
      |         'DelayLength', int2str(1));
      |     
      |     % Add bitslice
      |     add_block('hdlsllib/Logic and Bit Operations/Bit Slice',...
      |         [gcb, '/wr_bitslice'], 'Position',...
      |         [-65 180 25 220]);
      | 
      |     % Set bitslice parameters
      |     set_param([gcb, '/wr_bitslice'],...
      |         'lidx', int2str(ceil(log2(d)-1)));
      |     set_param([gcb, '/wr_bitslice'],...
      |         'ridx', int2str(log2(a(1))));
      |     
      |     % Add bitslice
      |     add_block('hdlsllib/Logic and Bit Operations/Bit Slice',...
      |         [gcb, '/rd_bitslice'], 'Position',...
      |         [-65 280 25 320]);
      | 
      |     % Set bitslice parameters
      |     set_param([gcb, '/rd_bitslice'],...
      |         'lidx', int2str(ceil(log2(d)-1)));
      |     set_param([gcb, '/rd_bitslice'],...
      |         'ridx', int2str(log2(a(1))));
      |     
      |     for i = 1:ceil(numbram)
      |         
      |         %%%%% Begin Adding Blocks %%%%%
      |         % Add Simple RAM
      |         add_block('hdlsllib/HDL RAMs/Simple Dual Port RAM',...
      |             [gcb, '/simple_ram_', int2str(i-1)], 'Position',...
      |             [635 0+600*y 635+200 400+600*y]);
      | 
      |         % Set RAM parameters
      |         set_param([gcb, '/simple_ram_', int2str(i-1)],...
      |             'ram_size', int2str(log2(a(1))));
      | 
      |         % Add compare to constant
      |         add_block('hdlsllib/Logic and Bit Operations/Compare To Constant',...
      |             [gcb, '/wr_cmp2const_', int2str(i-1)], 'Position',...
      |             [190 225+y*600 220 255+y*600]); 
      | 
      |         % Set compare to zero parameters
      |         set_param([gcb, '/wr_cmp2const_', int2str(i-1)],...
      |             'relop', '==');
      | 
      |         % Set compare to zero parameters
      |         set_param([gcb, '/wr_cmp2const_', int2str(i-1)],...
      |             'const', int2str(i-1));
      |         
      |         % Add compare to constant
      |         add_block('hdlsllib/Logic and Bit Operations/Compare To Constant',...
      |             [gcb, '/rd_cmp2const_', int2str(i-1)], 'Position',...
      |             [190 445+y*600 220 475+y*600]); 
      | 
      |         % Set compare to zero parameters
      |         set_param([gcb, '/rd_cmp2const_', int2str(i-1)],...
      |             'relop', '==');
      | 
      |         % Set compare to zero parameters
      |         set_param([gcb, '/rd_cmp2const_', int2str(i-1)],...
      |             'const', int2str(i-1));
      | 
      |         % Add and logic
      |         add_block('hdlsllib/Logic and Bit Operations/Logical Operator',...
      |             [gcb, '/and_', int2str(i-1)], 'Position',...
      |             [420 231+600*y 455 264+600*y]);
      | 
      |         % Set and logic parameters
      |         set_param([gcb, '/and_', int2str(i-1)],...
      |             'Operator', 'AND');
      | 
      |         % Add Switch
      |         add_block('hdlsllib/Signal Routing/Switch',...
      |             [gcb, '/switch_', int2str(i-1)], 'Position',...
      |             [685 -113+600*y 785 -37+600*y]);
      | 
      |         % Set switch parameters
      |         set_param([gcb, '/switch_', int2str(i-1)],...
      |             'Threshold', int2str(1));
      | 
      |         % Add Constant
      |         add_block('hdlsllib/Sources/Constant',...
      |             [gcb, '/constant_', int2str(i-1)], 'Position',...
      |             [425 -115+600*y 455 -85+600*y]);
      | 
      |         % Set Constant parameters
      |         set_param([gcb, '/constant_', int2str(i-1)],...
      |             'Value', int2str(i-1));
      |         set_param([gcb, '/constant_', int2str(i-1)],...
      |             'OutDataTypeStr', ['fixdt(0, ', int2str(ceil(numbram)), ', 0)']);   
      | 
      |         %%%%% Begin Wire Connections %%%%%        
      |         % Connect "wr_data" to "simple_ram_i"
      |         add_line(gcb, 'wr_data/1', ['simple_ram_', int2str(i-1), '/1'],...
      |             'autorouting','on');
      | 
      |         % Connect "wr_address" to "simple_ram_i"
      |         add_line(gcb, 'wr_address/1', ['simple_ram_', int2str(i-1), '/2'],...
      |             'autorouting','on');
      | 
      |         % Connect "rd_address" to "simple_ram_i"
      |         add_line(gcb, 'rd_address/1', ['simple_ram_', int2str(i-1), '/4'],...
      |             'autorouting','on');
      | 
      |         % Connect "constant_i" to "switch_i"
      |         add_line(gcb, ['constant_', int2str(i-1), '/1'], ['switch_', int2str(i-1), '/1'],...
      |             'autorouting','on');
      | 
      |         % Connect "zero" to "switch_i"
      |         add_line(gcb, 'zero/1', ['switch_', int2str(i-1), '/3'],...
      |             'autorouting','on');
      | 
      |         % Connect "switch_i" to "vector_concatenate"
      |         add_line(gcb, ['switch_', int2str(i-1), '/1'], ['vector_concatenate/', int2str(i)],...
      |             'autorouting','on');
      | 
      |         % Connect "rd_address" to "simple_ram_i"
      |         add_line(gcb, ['simple_ram_', int2str(i-1), '/1'],['multiport_switch/', int2str(i+1)],...
      |             'autorouting','on');
      | 
      |         % Connect "bitslice_i" to "wr_cmp2const_i"
      |         add_line(gcb, ['wr_bitslice/1'], ['wr_cmp2const_', int2str(i-1), '/1'],...
      |             'autorouting','on');
      |         
      |         % Connect "bitslice_i" to "rd_cmp2const_i"
      |         add_line(gcb, ['rd_bitslice/1'], ['rd_cmp2const_', int2str(i-1), '/1'],...
      |             'autorouting','on');
      | 
      |         % Connect "wr_en" to "and_i"
      |         add_line(gcb, ['wr_en/1'], ['and_', int2str(i-1), '/2'],...
      |             'autorouting','on');
      | 
      |         % Connect "and_i" to "simple_ram_0"
      |         add_line(gcb, ['and_', int2str(i-1), '/1'], ['simple_ram_', int2str(i-1), '/3'],...
      |             'autorouting','on');
      | 
      |         % Connect "wr_cmp2const_i" to "and_i"
      |         add_line(gcb, ['wr_cmp2const_', int2str(i-1), '/1'], ['and_', int2str(i-1), '/1'],...
      |             'autorouting','on');
      | 
      |         % Connect "rd_cmp2const_i" to "switch_i"
      |         add_line(gcb, ['rd_cmp2const_', int2str(i-1), '/1'], ['switch_', int2str(i-1), '/2'],...
      |             'autorouting','on');
      |          
      |         % Update coordinates
      |         y = y + 1;
      |         
      |     end
      |     
      |     % Connect "rd_addr" to "bitslice_i"
      |     add_line(gcb, ['rd_addr/1'], ['rd_bitslice/1'],...
      |         'autorouting','on');
      |     
      |     % Connect "wr_addr" to "bitslice_i"
      |     add_line(gcb, ['wr_addr/1'], ['wr_bitslice/1'],...
      |         'autorouting','on');
      |     
      |     % Connect "wr_addr" to "wr_address"
      |     add_line(gcb, 'wr_addr/1', ['wr_address', '/1'],...
      |         'autorouting','on');
      | 
      |     % Connect "rd_addr" to "rd_address"
      |     add_line(gcb, 'rd_addr/1', ['rd_address', '/1'],...
      |         'autorouting','on');
      | 
      |     % Connect "vector_concatenate" to "bitwise_or"
      |     add_line(gcb, ['vector_concatenate/1'], ['bitwise_or/1'],...
      |         'autorouting','on');
      | 
      |     % Connect "bitwise_or" to "delay"
      |     add_line(gcb, ['bitwise_or/1'], ['delay/1'],...
      |         'autorouting','on');
      | 
      |     % Connect "delay" to "multiport_switch"
      |     add_line(gcb, ['delay/1'], ['multiport_switch/1'],...
      |         'autorouting','on');
      | 
      |     % Connect "multiport_switch" to "rd_data"
      |     add_line(gcb, ['multiport_switch/1'], ['rd_data/1'],...
      |         'autorouting','on');
      |     
      | end
      | 
      | % If there is a half bram we must change a few parameters. Firstly, delete
      | % the write and read address lines. Then add bitslice blocks to reduce the
      | % address space in half. Connect rd_addr and wr_addr to the corresponding ports
      | % on the bram. Finally, change the address depth.
      | if halfbram
      |     
      |     if ceil(numbram) > 1
      |         
      |         % Delete lines
      |         delete_line(gcb, ['wr_address/1'], ['simple_ram_', int2str(i-1), '/2'])
      |         delete_line(gcb, ['rd_address/1'], ['simple_ram_', int2str(i-1), '/4'])
      |         
      |         % Write Address half ram Slice
      |         add_block('hdlsllib/Logic and Bit Operations/Bit Slice',...
      |                 [gcb, '/wr_address_hr'], 'Position',...
      |                 [160 130+(y-1)*600 250 170+(y-1)*600]);
      |         % Set bitslice parameters
      |         set_param([gcb, '/wr_address_hr'],...
      |             'lidx', int2str(log2(a(1))-2));
      |         set_param([gcb, '/wr_address_hr'],...
      |             'ridx', int2str(0));
      | 
      |         % Read Address half ram Slice
      |         add_block('hdlsllib/Logic and Bit Operations/Bit Slice',...
      |                 [gcb, '/rd_address_hr'], 'Position',...
      |                 [160 330+(y-1)*600 250 370+(y-1)*600]);
      |         % Set bitslice parameters
      |         set_param([gcb, '/rd_address_hr'],...
      |             'lidx', int2str(log2(a(1))-2));
      |         set_param([gcb, '/rd_address_hr'],...
      |             'ridx', int2str(0));
      | 
      |         % Connect "wr_addr" to "wr_address_hr"
      |         add_line(gcb, 'wr_addr/1', ['wr_address_hr', '/1'],...
      |             'autorouting','on');
      | 
      |         % Connect "rd_addr" to "rd_address_hr"
      |         add_line(gcb, 'rd_addr/1', ['rd_address_hr', '/1'],...
      |             'autorouting','on');
      | 
      |         % Connect "wr_address_hr" to "simple_ram_i"
      |         add_line(gcb, ['wr_address_hr', '/1'], ['simple_ram_', int2str(i-1), '/2'],...
      |             'autorouting','on');
      | 
      |         % Connect "rd_address_hr" to "simple_ram_i"
      |         add_line(gcb, ['rd_address_hr', '/1'], ['simple_ram_', int2str(i-1), '/4'],...
      |             'autorouting','on');
      | 
      |     else
      |         % Set bitslice parameters
      |         set_param([gcb, '/wr_address'],...
      |             'lidx', int2str(log2(a(1))-2));
      |         set_param([gcb, '/wr_address'],...
      |             'ridx', int2str(0));
      |         % Set bitslice parameters
      |         set_param([gcb, '/rd_address'],...
      |             'lidx', int2str(log2(a(1))-2));
      |         set_param([gcb, '/rd_address'],...
      |             'ridx', int2str(0));
      |         
      |     end
      |     
      |     % Update the ram parameters (address bits)
      |     set_param([gcb, '/simple_ram_', int2str(i-1)],...
      |         'ram_size', int2str(log2(a(1)/2)));
      |     
      | end
  rd_data : Outport
  wires:
  rd_addr/1 -> Simple Dual Port RAM Generator/4(rd_addr)
  wr_en/1 -> Simple Dual Port RAM Generator/3(wr_en)
  wr_addr/1 -> Simple Dual Port RAM Generator/2(wr_addr)
  wr_data/1 -> Simple Dual Port RAM Generator/1(wr_data)
  Simple Dual Port RAM Generator/1(rd_data) -> rd_data/1

== system gm_hybrid_lht_vnl/Hybrid LHT/Hybrid LHT Accumulator/Accumulator with Switches/Accumulator_instance10/Block RAM ==
  wr_data : Inport  OutDataTypeStr=fixdt(0, 36, 0)  PortDimensions=1  SampleTime=8.33333333333333e-09
  wr_addr : Inport  Port=2  OutDataTypeStr=fixdt(0, 11, 0)  PortDimensions=1  SampleTime=8.33333333333333e-09
  wr_en : Inport  Port=3  OutDataTypeStr=boolean  PortDimensions=1  SampleTime=8.33333333333333e-09
  rd_addr : Inport  Port=4  OutDataTypeStr=fixdt(0, 11, 0)  PortDimensions=1  SampleTime=8.33333333333333e-09
  Simple Dual Port RAM Generator : Subsystem  mask{b=double(36), d=double(1280), b_hidden=double(36), d_hidden=double(1280)}
      mask prompts: b "Data width:"; d "Depth:"
      mask init: same as gm_hybrid_lht_vnl/Hybrid LHT/Hybrid LHT Accumulator/Accumulator with Switches/Accumulator_instance1/Block RAM/Simple Dual Port RAM Generator
  rd_data : Outport
  wires:
  Simple Dual Port RAM Generator/1(rd_data) -> rd_data/1
  wr_data/1 -> Simple Dual Port RAM Generator/1(wr_data)
  wr_addr/1 -> Simple Dual Port RAM Generator/2(wr_addr)
  wr_en/1 -> Simple Dual Port RAM Generator/3(wr_en)
  rd_addr/1 -> Simple Dual Port RAM Generator/4(rd_addr)

== system gm_hybrid_lht_vnl/Hybrid LHT/Hybrid LHT Accumulator/Accumulator with Switches/Accumulator_instance11/Block RAM ==
  wr_data : Inport  OutDataTypeStr=fixdt(0, 36, 0)  PortDimensions=1  SampleTime=8.33333333333333e-09
  wr_addr : Inport  Port=2  OutDataTypeStr=fixdt(0, 11, 0)  PortDimensions=1  SampleTime=8.33333333333333e-09
  wr_en : Inport  Port=3  OutDataTypeStr=boolean  PortDimensions=1  SampleTime=8.33333333333333e-09
  rd_addr : Inport  Port=4  OutDataTypeStr=fixdt(0, 11, 0)  PortDimensions=1  SampleTime=8.33333333333333e-09
  Simple Dual Port RAM Generator : Subsystem  mask{b=double(36), d=double(1280), b_hidden=double(36), d_hidden=double(1280)}
      mask prompts: b "Data width:"; d "Depth:"
      mask init: same as gm_hybrid_lht_vnl/Hybrid LHT/Hybrid LHT Accumulator/Accumulator with Switches/Accumulator_instance1/Block RAM/Simple Dual Port RAM Generator
  rd_data : Outport
  wires:
  Simple Dual Port RAM Generator/1(rd_data) -> rd_data/1
  wr_data/1 -> Simple Dual Port RAM Generator/1(wr_data)
  wr_addr/1 -> Simple Dual Port RAM Generator/2(wr_addr)
  wr_en/1 -> Simple Dual Port RAM Generator/3(wr_en)
  rd_addr/1 -> Simple Dual Port RAM Generator/4(rd_addr)

== system gm_hybrid_lht_vnl/Hybrid LHT/Hybrid LHT Accumulator/Accumulator with Switches/Accumulator_instance12/Block RAM ==
  wr_data : Inport  OutDataTypeStr=fixdt(0, 36, 0)  PortDimensions=1  SampleTime=8.33333333333333e-09
  wr_addr : Inport  Port=2  OutDataTypeStr=fixdt(0, 11, 0)  PortDimensions=1  SampleTime=8.33333333333333e-09
  wr_en : Inport  Port=3  OutDataTypeStr=boolean  PortDimensions=1  SampleTime=8.33333333333333e-09
  rd_addr : Inport  Port=4  OutDataTypeStr=fixdt(0, 11, 0)  PortDimensions=1  SampleTime=8.33333333333333e-09
  Simple Dual Port RAM Generator : Subsystem  mask{b=double(36), d=double(1280), b_hidden=double(36), d_hidden=double(1280)}
      mask prompts: b "Data width:"; d "Depth:"
      mask init: same as gm_hybrid_lht_vnl/Hybrid LHT/Hybrid LHT Accumulator/Accumulator with Switches/Accumulator_instance1/Block RAM/Simple Dual Port RAM Generator
  rd_data : Outport
  wires:
  Simple Dual Port RAM Generator/1(rd_data) -> rd_data/1
  wr_data/1 -> Simple Dual Port RAM Generator/1(wr_data)
  wr_addr/1 -> Simple Dual Port RAM Generator/2(wr_addr)
  wr_en/1 -> Simple Dual Port RAM Generator/3(wr_en)
  rd_addr/1 -> Simple Dual Port RAM Generator/4(rd_addr)
